simulink model "Acseassignment"  (R2018a)
settings: Solver=VariableStepAuto  StartTime=0.0  StopTime=5  RelTol=1e-3
libraries: simulink x3
settings Model: Creator=krman  LastModifiedBy=krman

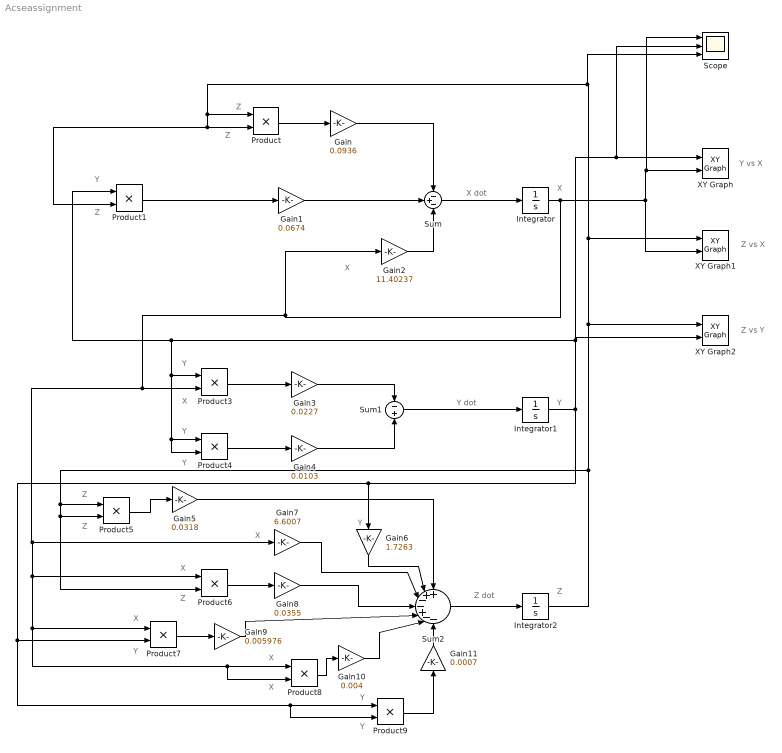
== system Acseassignment ==
  note: Z vs X
  note: Y vs X
  note: X
  note: X dot
  note: Y dot
  note: Y
  note: Z dot
  note: Z
  note: Z
  note: Z
  note: Z
  note: Y
  note: X
  note: Y
  note: X
  note: Y
  note: Y
  note: Z
  note: Z
  note: Y
  note: X
  note: X
  note: Z
  note: X
  note: Y
  note: X
  note: X
  note: Y
  note: Y
  note: Z vs Y
  Gain : Gain  Gain=0.0936
  Gain1 : Gain  Gain=0.0674
  Gain10 : Gain  Gain=0.004
  Gain11 : Gain  Gain=0.0007
  Gain2 : Gain  Gain=11.40237
  Gain3 : Gain  Gain=0.0227
  Gain4 : Gain  Gain=0.0103
  Gain5 : Gain  Gain=0.0318
  Gain6 : Gain  Gain=1.7263
  Gain7 : Gain  Gain=6.6007
  Gain8 : Gain  Gain=0.0355
  Gain9 : Gain  Gain=0.005976
  Integrator : Integrator  InitialCondition=1
  Integrator1 : Integrator  InitialCondition=1
  Integrator2 : Integrator  InitialCondition=1
  Product{,1,3..9} (9 alike) : Product
  Scope : Scope  NumInputPorts=3
  Sum : Sum  Inputs=-+-
  Sum1 : Sum  Inputs=-+
  Sum2 : Sum  Inputs=++--+--
  XY Graph : simulink/Sinks/XY Graph  xmin=-100  xmax=100  ymin=-100  ymax=100  st=0.0001
  XY Graph1 : simulink/Sinks/XY Graph  xmin=-100  xmax=100  ymin=-100  ymax=100  st=0.0001
  XY Graph2 : simulink/Sinks/XY Graph  xmin=-100  xmax=100  ymin=-100  ymax=100  st=0.0001
  wires:
  Sum1/1 -> Integrator1/1
  Product/1 -> Gain/1
  Product1/1 -> Gain1/1
  Product3/1 -> Gain3/1
  Product4/1 -> Gain4/1
  Product5/1 -> Gain5/1
  Product6/1 -> Gain8/1
  Product7/1 -> Gain9/1
  Product8/1 -> Gain10/1
  Product9/1 -> Gain11/1
  Sum/1 -> Integrator/1
  Sum2/1 -> Integrator2/1
  Integrator2/1 -> Product6/2, Product5/2, Product5/1, XY Graph2/1, XY Graph1/1, Scope/3, Product/1, Product1/2, Product/2
  Gain/1 -> Sum/1
  Gain1/1 -> Sum/2
  Integrator1/1 -> Product9/2, Product9/1, Product7/2, Gain6/1, XY Graph2/2, XY Graph/1, Scope/2, Product4/2, Product4/1, Product3/1, Product1/1
  Integrator/1 -> Gain2/1, Product8/2, Product8/1, Product7/1, Product6/1, Gain7/1, Product3/2, XY Graph1/2, XY Graph/2, Scope/1
  Gain2/1 -> Sum/3
  Gain3/1 -> Sum1/1
  Gain4/1 -> Sum1/2
  Gain5/1 -> Sum2/1
  Gain6/1 -> Sum2/2
  Gain7/1 -> Sum2/3
  Gain8/1 -> Sum2/4
  Gain9/1 -> Sum2/5
  Gain10/1 -> Sum2/6
  Gain11/1 -> Sum2/7
